simulink model "diagramaBloquesTruxal"  (R2024b)
settings: Solver=VariableStepAuto  StartTime=0.0  StopTime=10.0  RelTol=1e-3
settings Model: Creator=estel  LastModifiedBy=estel

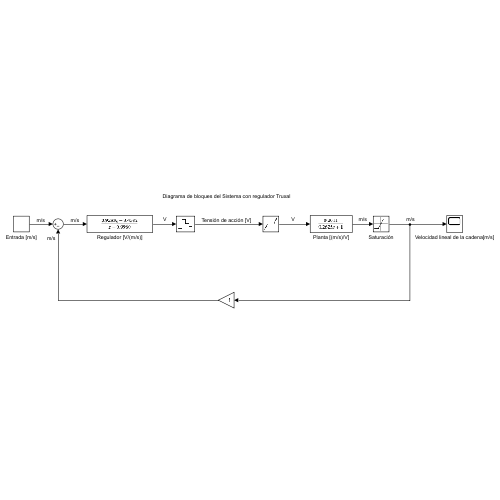
[thumbnail: Simulink's stored preview of the top-level diagram]
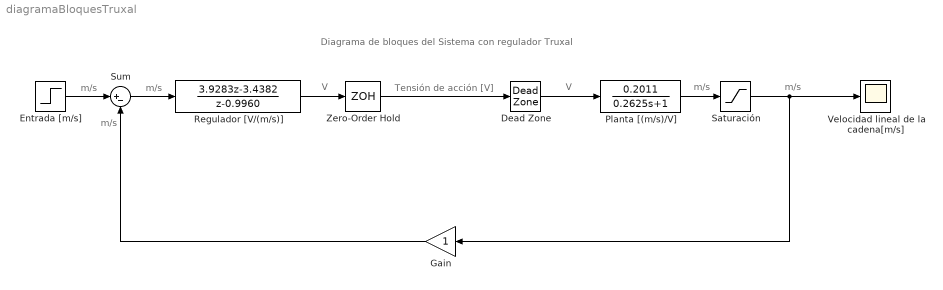
== system diagramaBloquesTruxal ==
  note: Diagrama de bloques del Sistema con regulador Truxal
  note: m/s
  note: m/s
  note: m/s
  note: m/s
  note: V
  note: Tensión de acción [V]
  note: m/s
  note: V
  Dead Zone : DeadZone
  Entrada [m/s] : Step  SampleTime=0.035
  Gain : Gain
  Planta [(m/s)/V] : TransferFcn  Numerator=[0.2011]  Denominator=[0.2625 1]
  Regulador [V/(m/s)] : DiscreteTransferFcn  Numerator=[3.9283 -3.4382]  Denominator=[1 -0.9960]
  Saturación : Saturate  UpperLimit=2.1098  LowerLimit=-2.1123
  Sum : Sum  Inputs=|+-
  Velocidad lineal de la cadena[m/s] : Scope
  Zero-Order Hold : ZeroOrderHold  SampleTime=-1
  wires:
  Entrada [m/s]/1 -> Sum/1
  Sum/1 -> Regulador [V/(m/s)]/1
  Gain/1 -> Sum/2
  Regulador [V/(m/s)]/1 -> Zero-Order Hold/1
  Planta [(m/s)/V]/1 -> Saturación/1
  Saturación/1 -> Gain/1, Velocidad lineal de la cadena[m/s]/1
  Dead Zone/1 -> Planta [(m/s)/V]/1
  Zero-Order Hold/1 -> Dead Zone/1
